simulink model "matrixconv1"  (Simulink 7.5)
settings: Solver=ode45  StartTime=0.0  StopTime=0.1  RelTol=1e-3
libraries: powerlib x46, powerlib_extras x4
settings Model: Creator=jeevitha  LastModifiedBy=Administrator
settings DebuggingCC: FcnCallInpInsideContextMsg=Enable All

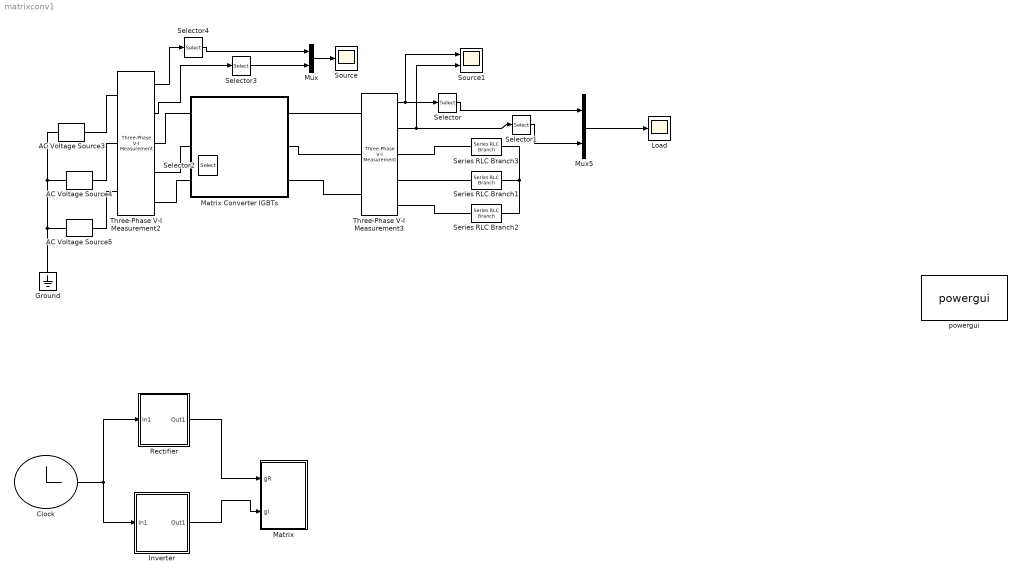
== system matrixconv1 ==
  AC Voltage Source3 : powerlib/Electrical Sources/AC Voltage Source  DialogController=POWERSYS.PowerSysDialog  SystemSampleTime=-1  Amplitude=230  Phase=0  Frequency=50  SampleTime=0  Measurements=None
  AC Voltage Source4 : powerlib/Electrical Sources/AC Voltage Source  DialogController=POWERSYS.PowerSysDialog  SystemSampleTime=-1  Amplitude=230  Phase=120  Frequency=50  SampleTime=0  Measurements=None
  AC Voltage Source5 : powerlib/Electrical Sources/AC Voltage Source  DialogController=POWERSYS.PowerSysDialog  SystemSampleTime=-1  Amplitude=230  Phase=-120  Frequency=50  SampleTime=0  Measurements=None
  Clock : Clock
  Ground : powerlib/Elements/Ground  DialogController=POWERSYS.PowerSysDialog  PhysicalDomain=powersysdomain  SubClassName=unknown  LeftPortType=p1  RightPortType=p1  LConnTagsString=a
  Inverter : Subsystem
  Load : Scope
      settings: TimeRange=0.012  YMin=-25  YMax=400  SaveName=vl
  Matrix : Subsystem
  Matrix Converter IGBTs : Subsystem
      mask Display:
      | plot([0 10],[0 0])
      | plot([0 10],[4 4])
      | plot([0 10],[8 8])
      | plot([10 11],[8 7],[11 12.5],[7 6.5],[12 13],[6 5])
      | plot([10 11]-4,[8 7],[11 12.5]-4,[7 6.5],[12 13]-4,[6 5])
      | plot([10 11]-8,[8 7],[11 12.5]-8,[7 6.5],[12 13]-8,[6 5])
      | plot([10 11],[8 7]-4,[11 12.5],[7 6.5]-4,[12 13],[6 5]-4)
      | plot([10 11]-4,[8 7]-4,[11 12.5]-4,[7 6.5]-4,[12 13]-4,[6 5]-4)
      | plot([10 11]-8,[8 7]-4,[11 12.5]-8,[7 6.5]-4,[12 13]-8,[6 5]-4)
      | plot([10 11],[8 7]-8,[11 12.5],[7 6.5]-8,[12 13],[6 5]-8)
      | plot([10 11]-4,[8 7]-8,[11 12.5]-4,[7 6.5]-8,[12 13]-4,[6 5]-8)
      | plot([10 11]-8,[8 7]-8,[11 12.5]-8,[7 6.5]-8,[12 13]-8,[6 5]-8)
      | plot([5 5],[-5 5])
      | plot([9 9],[-5 5])
      | plot([13 13],[-5 5])
      | plot(-2,-6,15,9)
      | plot([0 0],[-5 -2])
      | plot([0.5 0.5],[-5 -2])
      | plot([0.5 1.5],[-4 -5])
      | plot([0.5 1.5],[-3 -2])
      | plot([1.5 1.5],[-5 -6])
      | plot([1.5 1.5],[-2 -1])
      | plot([1 1.5],[-4.8 -5])
      | plot([1.3 1.5],[-4.4 -5])
      | plot([-0.5 0],[-5 -5])
  Mux : Mux  Inputs=2
  Mux5 : Mux  Inputs=2
  Rectifier : Subsystem
  Selector : Selector  InputPortWidth=3  IndexOptions=Index vector (dialog)  Indices=3  OutputSizes=1
  Selector1 : Selector  InputPortWidth=3  IndexOptions=Index vector (dialog)  Indices=3  OutputSizes=1
  Selector2 : Selector  InputPortWidth=3  IndexOptions=Index vector (dialog)  Indices=1  OutputSizes=1
  Selector3 : Selector  InputPortWidth=3  IndexOptions=Index vector (dialog)  Indices=1  OutputSizes=1
  Selector4 : Selector  InputPortWidth=3  IndexOptions=Index vector (dialog)  Indices=1  OutputSizes=1
  Series RLC Branch1 : powerlib/Elements/Series RLC Branch  DialogController=POWERSYS.PowerSysDialog  PhysicalDomain=powersysdomain  SubClassName=unknown  LeftPortType=p1  RightPortType=p1  LConnTagsString=__new0  RConnTagsString=__new0  BranchType=R  Resistance=2  Inductance=1e-3  SetiL0=off  InitialCurrent=0  Capacitance=[]  Setx0=off  InitialVoltage=0  Measurements=None
  Series RLC Branch2 : powerlib/Elements/Series RLC Branch  DialogController=POWERSYS.PowerSysDialog  PhysicalDomain=powersysdomain  SubClassName=unknown  LeftPortType=p1  RightPortType=p1  LConnTagsString=__new0  RConnTagsString=__new0  BranchType=R  Resistance=2  Inductance=1e-3  SetiL0=off  InitialCurrent=0  Capacitance=[]  Setx0=off  InitialVoltage=0  Measurements=None
  Series RLC Branch3 : powerlib/Elements/Series RLC Branch  DialogController=POWERSYS.PowerSysDialog  PhysicalDomain=powersysdomain  SubClassName=unknown  LeftPortType=p1  RightPortType=p1  LConnTagsString=__new0  RConnTagsString=__new0  BranchType=R  Resistance=2  Inductance=1e-3  SetiL0=off  InitialCurrent=0  Capacitance=[]  Setx0=off  InitialVoltage=0  Measurements=None
  Source : Scope
      settings: TimeRange=0.09  YMin=-100  YMax=100  SaveName=vl1
  Source1 : Scope  NumInputPorts=2
      settings: TimeRange=0.09  YMin=-100~-5  YMax=100~5  SaveName=vl2
  Three-Phase V-I Measurement2 : powerlib/Measurements/Three-Phase V-I Measurement  DialogController=POWERSYS.PowerSysDialog  SystemSampleTime=-1  VoltageMeasurement=phase-to-ground  SetLabelV=off  LabelV=Vabc  Vpu=off  VpuLL=off  CurrentMeasurement=yes  SetLabelI=off  LabelI=Iabc  Ipu=off  Pbase=100e6  Vbase=500e3  OutputType=Complex  PhasorSimulation=off  PSBequivalent=0
      link override Model/VI/Ia: GotoTag=LibraryTag_Ia
      link override Model/VI/Ib: GotoTag=LibraryTag_Ib
      link override Model/VI/Ic: GotoTag=LibraryTag_Ic
      link override Model/VI/Va: GotoTag=LibraryTag_Va
      link override Model/VI/Vb: GotoTag=LibraryTag_Vb
      link override Model/VI/Vc: GotoTag=LibraryTag_Vc
  Three-Phase V-I Measurement3 : powerlib/Measurements/Three-Phase V-I Measurement  DialogController=POWERSYS.PowerSysDialog  SystemSampleTime=-1  VoltageMeasurement=phase-to-phase  SetLabelV=off  LabelV=Vabc  Vpu=off  VpuLL=off  CurrentMeasurement=yes  SetLabelI=off  LabelI=Iabc  Ipu=off  Pbase=100e6  Vbase=500e3  OutputType=Complex  PhasorSimulation=off  PSBequivalent=0
      link override Model/VI/Ia: GotoTag=LibraryTag_Ia
      link override Model/VI/Ib: GotoTag=LibraryTag_Ib
      link override Model/VI/Ic: GotoTag=LibraryTag_Ic
      link override Model/VI/Va: GotoTag=LibraryTag_Va
      link override Model/VI/Vb: GotoTag=LibraryTag_Vb
      link override Model/VI/Vc: GotoTag=LibraryTag_Vc
  powergui : powerlib/powergui  Priority=1  SystemSampleTime=-1  SimulationMode=Discrete  SampleTime=((2e-4)/8)/100  frequency=60  SPID=off  DisableSnubberDevices=off  DisableRonSwitches=off  DisableVfSwitches=off  SwTol=0  Interpol=off  frequencyindice=0  echomessages=off  HookPort=off  DisplayEquations=off  FunctionMessages=off  EnableUseOfTLC=off  x0status=blocks  RestoreLinks=warning  ResistiveCurrentMeasurement=off  Frange=[0:2:500]  Ylog=off  Xlog=on  ShowGrid=off  save=off  variable=ZData  structure=ScopeData1  ZoomFFT=off  StartTime=0.02  cycles=1  DisplayStyle=3  fundamental=50  FreqAxis=off  MaxFrequency=1000  frequencyindicesteady=0  RmsSteady=2  display=off  Ts=0  methode=off
  wires:
  Clock/1 -> Rectifier/1(In1), Inverter/1(In1)
  Rectifier/1(Out1) -> Matrix/1(gR)
  Inverter/1(Out1) -> Matrix/2(gI)
  Three-Phase V-I Measurement3/1 -> Selector/1, Source1/1
  Three-Phase V-I Measurement3/2 -> Selector1/1, Source1/2
  Selector/1 -> Mux5/1
  Selector1/1 -> Mux5/2
  Mux5/1 -> Load/1
  Three-Phase V-I Measurement2/2 -> Selector3/1
  Three-Phase V-I Measurement2/1 -> Selector4/1
  Mux/1 -> Source/1
  Selector4/1 -> Mux/1
  Selector3/1 -> Mux/2
  connections:
  Series RLC Branch2/RConn1 -- Series RLC Branch3/RConn1 -- Series RLC Branch1/RConn1
  AC Voltage Source5/LConn1 -- Ground/LConn1 -- AC Voltage Source3/LConn1 -- AC Voltage Source4/LConn1
  Three-Phase V-I Measurement3/RConn1 -- Series RLC Branch3/LConn1
  Matrix Converter IGBTs/RConn1 -- Three-Phase V-I Measurement3/LConn1
  Matrix Converter IGBTs/RConn2 -- Three-Phase V-I Measurement3/LConn2
  Matrix Converter IGBTs/RConn3 -- Three-Phase V-I Measurement3/LConn3
  Three-Phase V-I Measurement3/RConn2 -- Series RLC Branch1/LConn1
  Three-Phase V-I Measurement3/RConn3 -- Series RLC Branch2/LConn1
  AC Voltage Source3/RConn1 -- Three-Phase V-I Measurement2/LConn1
  AC Voltage Source4/RConn1 -- Three-Phase V-I Measurement2/LConn2
  Three-Phase V-I Measurement2/LConn3 -- AC Voltage Source5/RConn1
  Three-Phase V-I Measurement2/RConn1 -- Matrix Converter IGBTs/LConn1
  Three-Phase V-I Measurement2/RConn2 -- Matrix Converter IGBTs/LConn2
  Three-Phase V-I Measurement2/RConn3 -- Matrix Converter IGBTs/LConn3

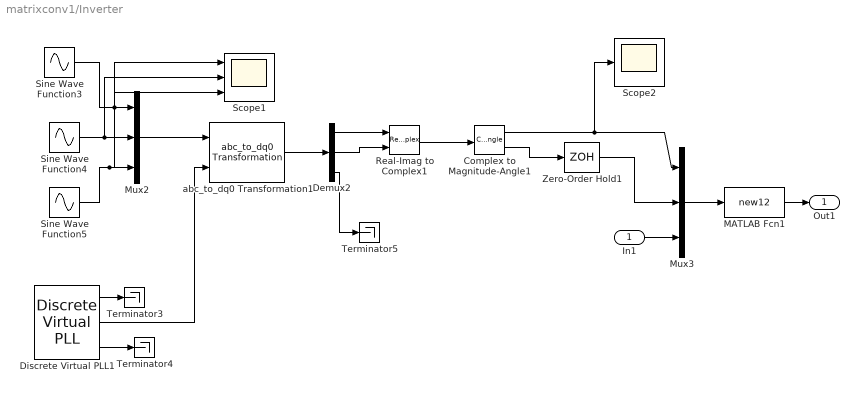
== system matrixconv1/Inverter ==
  In1 : Inport
  Complex to Magnitude-Angle1 : ComplexToMagnitudeAngle  SampleTime=((2e-4)/8)/100
  Demux2 : Demux  Outputs=3
  Discrete Virtual PLL1 : powerlib_extras/Discrete  Control Blocks/Discrete Virtual PLL  DialogController=POWERSYS.PowerSysDialog  SystemSampleTime=-1  Freq=25  Phase=0  Ts=((2e-4)/8)/100
  MATLAB Fcn1 : MATLABFcn  MATLABFcn=new12  OutputDimensions=6  SampleTime=((2e-4)/8)/100
  Mux2 : Mux  Inputs=3
  Mux3 : Mux  Inputs=3
  Real-Imag to Complex1 : RealImagToComplex  SampleTime=((2e-4)/8)/100
  Scope1 : Scope  NumInputPorts=3
      settings: YMin=0~175~-217  YMax=42.5~200~-199
  Scope2 : Scope
      settings: YMin=0  YMax=42.5  SaveName=ScopeData2
  Sine Wave Function3 : Sin  Amplitude=230  Bias=0  Frequency=2*pi*25  Phase=-(pi/6)  Samples=10  Offset=0
  Sine Wave Function4 : Sin  Amplitude=230  Bias=0  Frequency=2*pi*25  Phase=(2*pi/3)-(pi/6)  Samples=10  Offset=0
  Sine Wave Function5 : Sin  Amplitude=230  Bias=0  Frequency=2*pi*25  Phase=(4*pi/3)-(pi/6)  Samples=10  Offset=0
  Terminator3 : Terminator
  Terminator4 : Terminator
  Terminator5 : Terminator
  Zero-Order Hold1 : ZeroOrderHold  SampleTime=.0001005
  abc_to_dq0 Transformation1 : powerlib_extras/Measurements/abc_to_dq0 Transformation  DialogController=POWERSYS.PowerSysDialog  SystemSampleTime=-1
  Out1 : Outport
  wires:
  Discrete Virtual PLL1/1 -> Terminator3/1
  Discrete Virtual PLL1/3 -> Terminator4/1
  Sine Wave Function3/1 -> Mux2/1, Scope1/1
  Sine Wave Function4/1 -> Mux2/2, Scope1/2
  Sine Wave Function5/1 -> Mux2/3, Scope1/3
  Mux2/1 -> abc_to_dq0 Transformation1/1
  Discrete Virtual PLL1/2 -> abc_to_dq0 Transformation1/2
  abc_to_dq0 Transformation1/1 -> Demux2/1
  Demux2/3 -> Terminator5/1
  Demux2/1 -> Real-Imag to Complex1/1
  Demux2/2 -> Real-Imag to Complex1/2
  Real-Imag to Complex1/1 -> Complex to Magnitude-Angle1/1
  Complex to Magnitude-Angle1/2 -> Zero-Order Hold1/1
  Complex to Magnitude-Angle1/1 -> Mux3/1, Scope2/1
  Zero-Order Hold1/1 -> Mux3/2
  Mux3/1 -> MATLAB Fcn1/1
  In1/1 -> Mux3/3
  MATLAB Fcn1/1 -> Out1/1

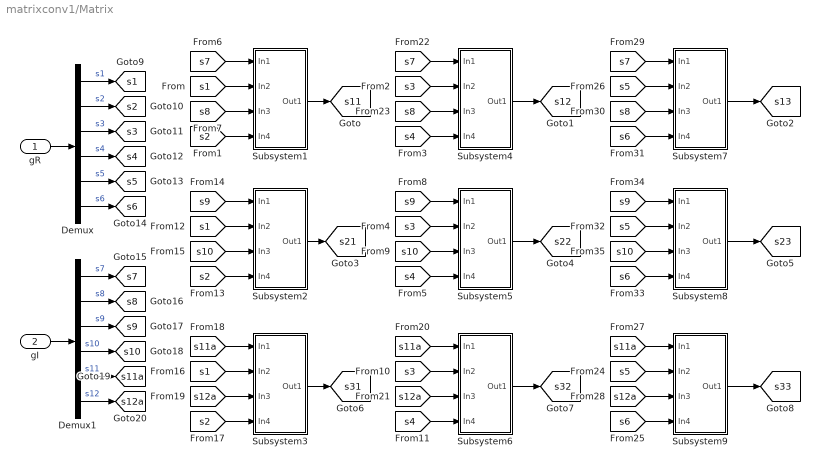
== system matrixconv1/Matrix ==
  gR : Inport
  gI : Inport  Port=2
  Demux : Demux  Outputs=6
  Demux1 : Demux  Outputs=6
  Subsystem1 : Subsystem
  Subsystem2 : Subsystem
  Subsystem3 : Subsystem
  Subsystem4 : Subsystem
  Subsystem5 : Subsystem
  Subsystem6 : Subsystem
  Subsystem7 : Subsystem
  Subsystem8 : Subsystem
  Subsystem9 : Subsystem
  tag scope: s10=global, s11=global, s11a=global, s12=global, s12a=global, s13=global, s1=global, s21=global, s22=global, s23=global, s2=global, s31=global, s32=global, s33=global, s3=global, s4=global, s5=global, s6=global, s7=global, s8=global, s9=global
  wires:
  Demux/4 -> [s4]  "s4"
  gR/1 -> Demux/1
  gI/1 -> Demux1/1
  Demux/1 -> [s1]  "s1"
  Demux1/1 -> [s7]  "s7"
  Demux/2 -> [s2]  "s2"
  Demux/3 -> [s3]  "s3"
  Demux/5 -> [s5]  "s5"
  Demux/6 -> [s6]  "s6"
  [s7] -> Subsystem1/1(In1)
  [s1] -> Subsystem1/2(In2)
  [s8] -> Subsystem1/3(In3)
  [s2] -> Subsystem1/4(In4)
  [s9] -> Subsystem2/1(In1)
  [s1] -> Subsystem2/2(In2)
  [s10] -> Subsystem2/3(In3)
  [s2] -> Subsystem2/4(In4)
  [s11a] -> Subsystem3/1(In1)
  [s1] -> Subsystem3/2(In2)
  [s12a] -> Subsystem3/3(In3)
  [s2] -> Subsystem3/4(In4)
  [s7] -> Subsystem4/1(In1)
  [s3] -> Subsystem4/2(In2)
  [s8] -> Subsystem4/3(In3)
  [s4] -> Subsystem4/4(In4)
  [s9] -> Subsystem5/1(In1)
  [s3] -> Subsystem5/2(In2)
  [s10] -> Subsystem5/3(In3)
  [s4] -> Subsystem5/4(In4)
  [s11a] -> Subsystem6/1(In1)
  [s3] -> Subsystem6/2(In2)
  [s12a] -> Subsystem6/3(In3)
  [s4] -> Subsystem6/4(In4)
  [s7] -> Subsystem7/1(In1)
  [s5] -> Subsystem7/2(In2)
  [s8] -> Subsystem7/3(In3)
  [s6] -> Subsystem7/4(In4)
  [s9] -> Subsystem8/1(In1)
  [s5] -> Subsystem8/2(In2)
  [s10] -> Subsystem8/3(In3)
  [s6] -> Subsystem8/4(In4)
  [s11a] -> Subsystem9/1(In1)
  [s5] -> Subsystem9/2(In2)
  [s12a] -> Subsystem9/3(In3)
  [s6] -> Subsystem9/4(In4)
  Subsystem1/1(Out1) -> [s11]
  Subsystem4/1(Out1) -> [s12]
  Subsystem7/1(Out1) -> [s13]
  Subsystem2/1(Out1) -> [s21]
  Subsystem5/1(Out1) -> [s22]
  Subsystem8/1(Out1) -> [s23]
  Subsystem3/1(Out1) -> [s31]
  Subsystem6/1(Out1) -> [s32]
  Subsystem9/1(Out1) -> [s33]
  Demux1/2 -> [s8]  "s8"
  Demux1/3 -> [s9]  "s9"
  Demux1/4 -> [s10]  "s10"
  Demux1/5 -> [s11a]  "s11"
  Demux1/6 -> [s12a]  "s12"

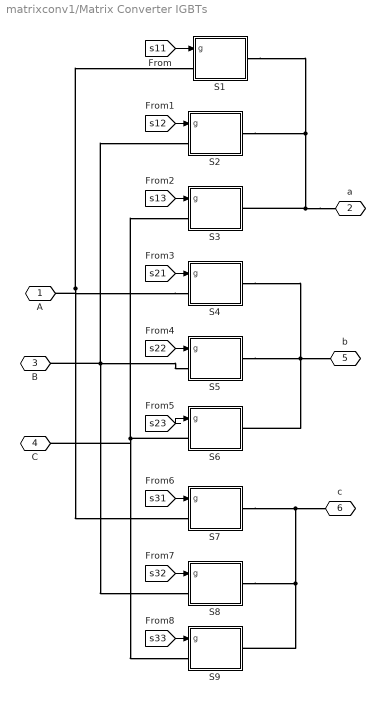
== system matrixconv1/Matrix Converter IGBTs ==
  S1 : Subsystem
  S2 : Subsystem
  S3 : Subsystem
  S4 : Subsystem
  S5 : Subsystem
  S6 : Subsystem
  S7 : Subsystem
  S8 : Subsystem
  S9 : Subsystem
  A : PMIOPort  Port=1  Side=Left
  a : PMIOPort  Port=2  Side=Right
  B : PMIOPort  Port=3  Side=Left
  C : PMIOPort  Port=4  Side=Left
  b : PMIOPort  Port=5  Side=Right
  c : PMIOPort  Port=6  Side=Right
  wires:
  [s11] -> S1/1(g)
  [s12] -> S2/1(g)
  [s13] -> S3/1(g)
  [s21] -> S4/1(g)
  [s22] -> S5/1(g)
  [s23] -> S6/1(g)
  [s31] -> S7/1(g)
  [s32] -> S8/1(g)
  [s33] -> S9/1(g)
  connections:
  S4/LConn1 -- A/RConn1 -- S1/LConn1 -- S7/LConn1
  a/RConn1 -- S2/RConn1 -- S1/RConn1 -- S3/RConn1
  S5/LConn1 -- S2/LConn1 -- B/RConn1 -- S8/LConn1
  S6/LConn1 -- S3/LConn1 -- C/RConn1 -- S9/LConn1
  S5/RConn1 -- S4/RConn1 -- b/RConn1 -- S6/RConn1
  S8/RConn1 -- S7/RConn1 -- c/RConn1 -- S9/RConn1

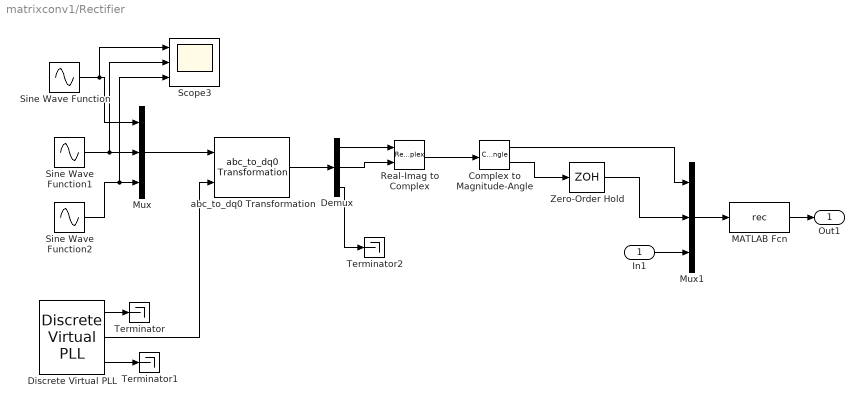
== system matrixconv1/Rectifier ==
  In1 : Inport
  Complex to Magnitude-Angle : ComplexToMagnitudeAngle  SampleTime=((2e-4)/8)/100
  Demux : Demux  Outputs=3
  Discrete Virtual PLL : powerlib_extras/Discrete  Control Blocks/Discrete Virtual PLL  DialogController=POWERSYS.PowerSysDialog  SystemSampleTime=-1  Freq=25  Phase=0  Ts=((2e-4)/8)/100
  MATLAB Fcn : MATLABFcn  MATLABFcn=rec  OutputDimensions=6  SampleTime=((2e-4)/8)/100
  Mux : Mux  Inputs=3
  Mux1 : Mux  Inputs=3
  Real-Imag to Complex : RealImagToComplex  SampleTime=((2e-4)/8)/100
  Scope3 : Scope  NumInputPorts=3
      settings: YMin=-182.5~213~-82.5  YMax=-145~227~-32.5
  Sine Wave Function : Sin  Amplitude=230  Bias=0  Frequency=2*pi*25  Phase=+(pi/6)  Samples=10  Offset=0
  Sine Wave Function1 : Sin  Amplitude=230  Bias=0  Frequency=2*pi*25  Phase=(2*pi/3)+(pi/6)  Samples=10  Offset=0
  Sine Wave Function2 : Sin  Amplitude=230  Bias=0  Frequency=2*pi*25  Phase=(4*pi/3)+(pi/6)  Samples=10  Offset=0
  Terminator : Terminator
  Terminator1 : Terminator
  Terminator2 : Terminator
  Zero-Order Hold : ZeroOrderHold  SampleTime=.0001005
  abc_to_dq0 Transformation : powerlib_extras/Measurements/abc_to_dq0 Transformation  DialogController=POWERSYS.PowerSysDialog  SystemSampleTime=-1
  Out1 : Outport
  wires:
  Discrete Virtual PLL/1 -> Terminator/1
  Discrete Virtual PLL/3 -> Terminator1/1
  Sine Wave Function/1 -> Mux/1, Scope3/1
  Sine Wave Function1/1 -> Mux/2, Scope3/2
  Sine Wave Function2/1 -> Mux/3, Scope3/3
  Mux/1 -> abc_to_dq0 Transformation/1
  Discrete Virtual PLL/2 -> abc_to_dq0 Transformation/2
  abc_to_dq0 Transformation/1 -> Demux/1
  Demux/3 -> Terminator2/1
  Demux/1 -> Real-Imag to Complex/1
  Demux/2 -> Real-Imag to Complex/2
  Real-Imag to Complex/1 -> Complex to Magnitude-Angle/1
  Complex to Magnitude-Angle/2 -> Zero-Order Hold/1
  Complex to Magnitude-Angle/1 -> Mux1/1
  Zero-Order Hold/1 -> Mux1/2
  Mux1/1 -> MATLAB Fcn/1
  In1/1 -> Mux1/3
  MATLAB Fcn/1 -> Out1/1

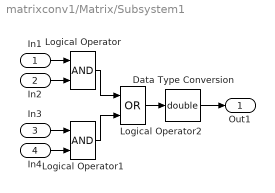
== system matrixconv1/Matrix/Subsystem1 ==
  In1 : Inport
  In2 : Inport  Port=2
  In3 : Inport  Port=3
  In4 : Inport  Port=4
  Data Type Conversion : DataTypeConversion  OutDataTypeMode=double  OutDataTypeStr=double
  Logical Operator : Logic  AllPortsSameDT=off  OutDataTypeMode=boolean  OutDataTypeStr=boolean
  Logical Operator1 : Logic  AllPortsSameDT=off  OutDataTypeMode=boolean  OutDataTypeStr=boolean
  Logical Operator2 : Logic  Operator=OR  AllPortsSameDT=off  OutDataTypeMode=boolean  OutDataTypeStr=boolean
  Out1 : Outport
  wires:
  In4/1 -> Logical Operator1/2
  In3/1 -> Logical Operator1/1
  Logical Operator2/1 -> Data Type Conversion/1
  In2/1 -> Logical Operator/2
  In1/1 -> Logical Operator/1
  Logical Operator1/1 -> Logical Operator2/2
  Logical Operator/1 -> Logical Operator2/1
  Data Type Conversion/1 -> Out1/1

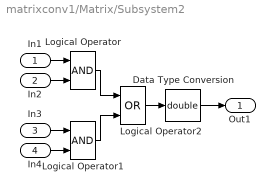
== system matrixconv1/Matrix/Subsystem2 ==
  In1 : Inport
  In2 : Inport  Port=2
  In3 : Inport  Port=3
  In4 : Inport  Port=4
  Data Type Conversion : DataTypeConversion  OutDataTypeMode=double  OutDataTypeStr=double
  Logical Operator : Logic  AllPortsSameDT=off  OutDataTypeMode=boolean  OutDataTypeStr=boolean
  Logical Operator1 : Logic  AllPortsSameDT=off  OutDataTypeMode=boolean  OutDataTypeStr=boolean
  Logical Operator2 : Logic  Operator=OR  AllPortsSameDT=off  OutDataTypeMode=boolean  OutDataTypeStr=boolean
  Out1 : Outport
  wires:
  In4/1 -> Logical Operator1/2
  In3/1 -> Logical Operator1/1
  Logical Operator2/1 -> Data Type Conversion/1
  In2/1 -> Logical Operator/2
  In1/1 -> Logical Operator/1
  Logical Operator1/1 -> Logical Operator2/2
  Logical Operator/1 -> Logical Operator2/1
  Data Type Conversion/1 -> Out1/1

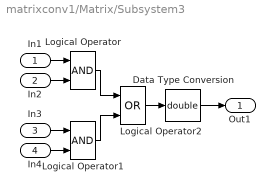
== system matrixconv1/Matrix/Subsystem3 ==
  In1 : Inport
  In2 : Inport  Port=2
  In3 : Inport  Port=3
  In4 : Inport  Port=4
  Data Type Conversion : DataTypeConversion  OutDataTypeMode=double  OutDataTypeStr=double
  Logical Operator : Logic  AllPortsSameDT=off  OutDataTypeMode=boolean  OutDataTypeStr=boolean
  Logical Operator1 : Logic  AllPortsSameDT=off  OutDataTypeMode=boolean  OutDataTypeStr=boolean
  Logical Operator2 : Logic  Operator=OR  AllPortsSameDT=off  OutDataTypeMode=boolean  OutDataTypeStr=boolean
  Out1 : Outport
  wires:
  In4/1 -> Logical Operator1/2
  In3/1 -> Logical Operator1/1
  Logical Operator2/1 -> Data Type Conversion/1
  In2/1 -> Logical Operator/2
  In1/1 -> Logical Operator/1
  Logical Operator1/1 -> Logical Operator2/2
  Logical Operator/1 -> Logical Operator2/1
  Data Type Conversion/1 -> Out1/1

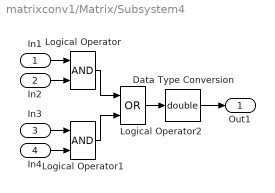
== system matrixconv1/Matrix/Subsystem4 ==
  In1 : Inport
  In2 : Inport  Port=2
  In3 : Inport  Port=3
  In4 : Inport  Port=4
  Data Type Conversion : DataTypeConversion  OutDataTypeMode=double  OutDataTypeStr=double
  Logical Operator : Logic  AllPortsSameDT=off  OutDataTypeMode=boolean  OutDataTypeStr=boolean
  Logical Operator1 : Logic  AllPortsSameDT=off  OutDataTypeMode=boolean  OutDataTypeStr=boolean
  Logical Operator2 : Logic  Operator=OR  AllPortsSameDT=off  OutDataTypeMode=boolean  OutDataTypeStr=boolean
  Out1 : Outport
  wires:
  In4/1 -> Logical Operator1/2
  In3/1 -> Logical Operator1/1
  Logical Operator2/1 -> Data Type Conversion/1
  In2/1 -> Logical Operator/2
  In1/1 -> Logical Operator/1
  Logical Operator1/1 -> Logical Operator2/2
  Logical Operator/1 -> Logical Operator2/1
  Data Type Conversion/1 -> Out1/1

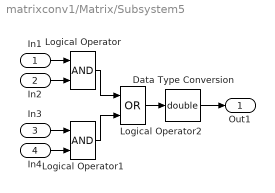
== system matrixconv1/Matrix/Subsystem5 ==
  In1 : Inport
  In2 : Inport  Port=2
  In3 : Inport  Port=3
  In4 : Inport  Port=4
  Data Type Conversion : DataTypeConversion  OutDataTypeMode=double  OutDataTypeStr=double
  Logical Operator : Logic  AllPortsSameDT=off  OutDataTypeMode=boolean  OutDataTypeStr=boolean
  Logical Operator1 : Logic  AllPortsSameDT=off  OutDataTypeMode=boolean  OutDataTypeStr=boolean
  Logical Operator2 : Logic  Operator=OR  AllPortsSameDT=off  OutDataTypeMode=boolean  OutDataTypeStr=boolean
  Out1 : Outport
  wires:
  In4/1 -> Logical Operator1/2
  In3/1 -> Logical Operator1/1
  Logical Operator2/1 -> Data Type Conversion/1
  In2/1 -> Logical Operator/2
  In1/1 -> Logical Operator/1
  Logical Operator1/1 -> Logical Operator2/2
  Logical Operator/1 -> Logical Operator2/1
  Data Type Conversion/1 -> Out1/1

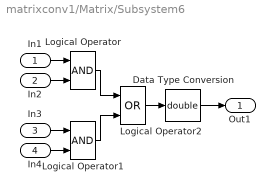
== system matrixconv1/Matrix/Subsystem6 ==
  In1 : Inport
  In2 : Inport  Port=2
  In3 : Inport  Port=3
  In4 : Inport  Port=4
  Data Type Conversion : DataTypeConversion  OutDataTypeMode=double  OutDataTypeStr=double
  Logical Operator : Logic  AllPortsSameDT=off  OutDataTypeMode=boolean  OutDataTypeStr=boolean
  Logical Operator1 : Logic  AllPortsSameDT=off  OutDataTypeMode=boolean  OutDataTypeStr=boolean
  Logical Operator2 : Logic  Operator=OR  AllPortsSameDT=off  OutDataTypeMode=boolean  OutDataTypeStr=boolean
  Out1 : Outport
  wires:
  In4/1 -> Logical Operator1/2
  In3/1 -> Logical Operator1/1
  Logical Operator2/1 -> Data Type Conversion/1
  In2/1 -> Logical Operator/2
  In1/1 -> Logical Operator/1
  Logical Operator1/1 -> Logical Operator2/2
  Logical Operator/1 -> Logical Operator2/1
  Data Type Conversion/1 -> Out1/1

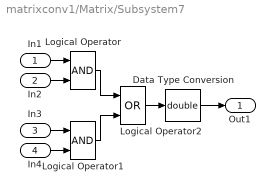
== system matrixconv1/Matrix/Subsystem7 ==
  In1 : Inport
  In2 : Inport  Port=2
  In3 : Inport  Port=3
  In4 : Inport  Port=4
  Data Type Conversion : DataTypeConversion  OutDataTypeMode=double  OutDataTypeStr=double
  Logical Operator : Logic  AllPortsSameDT=off  OutDataTypeMode=boolean  OutDataTypeStr=boolean
  Logical Operator1 : Logic  AllPortsSameDT=off  OutDataTypeMode=boolean  OutDataTypeStr=boolean
  Logical Operator2 : Logic  Operator=OR  AllPortsSameDT=off  OutDataTypeMode=boolean  OutDataTypeStr=boolean
  Out1 : Outport
  wires:
  In4/1 -> Logical Operator1/2
  In3/1 -> Logical Operator1/1
  Logical Operator2/1 -> Data Type Conversion/1
  In2/1 -> Logical Operator/2
  In1/1 -> Logical Operator/1
  Logical Operator1/1 -> Logical Operator2/2
  Logical Operator/1 -> Logical Operator2/1
  Data Type Conversion/1 -> Out1/1

== system matrixconv1/Matrix/Subsystem8 ==
  In1 : Inport
  In2 : Inport  Port=2
  In3 : Inport  Port=3
  In4 : Inport  Port=4
  Data Type Conversion : DataTypeConversion  OutDataTypeMode=double  OutDataTypeStr=double
  Logical Operator : Logic  AllPortsSameDT=off  OutDataTypeMode=boolean  OutDataTypeStr=boolean
  Logical Operator1 : Logic  AllPortsSameDT=off  OutDataTypeMode=boolean  OutDataTypeStr=boolean
  Logical Operator2 : Logic  Operator=OR  AllPortsSameDT=off  OutDataTypeMode=boolean  OutDataTypeStr=boolean
  Out1 : Outport
  wires:
  In4/1 -> Logical Operator1/2
  In3/1 -> Logical Operator1/1
  Logical Operator2/1 -> Data Type Conversion/1
  In2/1 -> Logical Operator/2
  In1/1 -> Logical Operator/1
  Logical Operator1/1 -> Logical Operator2/2
  Logical Operator/1 -> Logical Operator2/1
  Data Type Conversion/1 -> Out1/1

== system matrixconv1/Matrix/Subsystem9 ==
  In1 : Inport
  In2 : Inport  Port=2
  In3 : Inport  Port=3
  In4 : Inport  Port=4
  Data Type Conversion : DataTypeConversion  OutDataTypeMode=double  OutDataTypeStr=double
  Logical Operator : Logic  AllPortsSameDT=off  OutDataTypeMode=boolean  OutDataTypeStr=boolean
  Logical Operator1 : Logic  AllPortsSameDT=off  OutDataTypeMode=boolean  OutDataTypeStr=boolean
  Logical Operator2 : Logic  Operator=OR  AllPortsSameDT=off  OutDataTypeMode=boolean  OutDataTypeStr=boolean
  Out1 : Outport
  wires:
  In4/1 -> Logical Operator1/2
  In3/1 -> Logical Operator1/1
  Logical Operator2/1 -> Data Type Conversion/1
  In2/1 -> Logical Operator/2
  In1/1 -> Logical Operator/1
  Logical Operator1/1 -> Logical Operator2/2
  Logical Operator/1 -> Logical Operator2/1
  Data Type Conversion/1 -> Out1/1

== system matrixconv1/Matrix Converter IGBTs/S1 ==
  g : Inport
  Diode : powerlib/Power Electronics/Diode  DialogController=POWERSYS.PowerSysDialog  SystemSampleTime=-1  Ron=0.001  Lon=0  Vf=0  IC=0  UseSnubber=off  Rs=1e4  Cs=250e-9  Measurements=off
  Diode1 : powerlib/Power Electronics/Diode  DialogController=POWERSYS.PowerSysDialog  SystemSampleTime=-1  Ron=0.001  Lon=0  Vf=0  IC=0  UseSnubber=off  Rs=1e4  Cs=250e-9  Measurements=off
  IGBT1 : powerlib/Power Electronics/IGBT  DialogController=POWERSYS.PowerSysDialog  SystemSampleTime=-1  Ron=0.001  Lon=0  Vf=1  Tf=1e-6  Tt=2e-6  IC=0  Rs=1e5  Cs=inf  Measurements=off
  IGBT2 : powerlib/Power Electronics/IGBT  DialogController=POWERSYS.PowerSysDialog  SystemSampleTime=-1  Ron=0.001  Lon=0  Vf=1  Tf=1e-6  Tt=2e-6  IC=0  Rs=1e5  Cs=inf  Measurements=off
  + : PMIOPort  Port=1  Side=Left
  - : PMIOPort  Port=2  Side=Right
  wires:
  g/1 -> IGBT1/1, IGBT2/1
  connections:
  Diode1/LConn1 -- Diode/LConn1 -- IGBT1/RConn1 -- IGBT2/RConn1
  -/RConn1 -- Diode1/RConn1 -- IGBT1/LConn1
  +/RConn1 -- Diode/RConn1 -- IGBT2/LConn1

== system matrixconv1/Matrix Converter IGBTs/S2 ==
  g : Inport
  Diode : powerlib/Power Electronics/Diode  DialogController=POWERSYS.PowerSysDialog  SystemSampleTime=-1  Ron=0.001  Lon=0  Vf=0  IC=0  UseSnubber=off  Rs=1e4  Cs=250e-9  Measurements=off
  Diode1 : powerlib/Power Electronics/Diode  DialogController=POWERSYS.PowerSysDialog  SystemSampleTime=-1  Ron=0.001  Lon=0  Vf=0  IC=0  UseSnubber=off  Rs=1e4  Cs=250e-9  Measurements=off
  IGBT1 : powerlib/Power Electronics/IGBT  DialogController=POWERSYS.PowerSysDialog  SystemSampleTime=-1  Ron=0.001  Lon=0  Vf=1  Tf=1e-6  Tt=2e-6  IC=0  Rs=1e5  Cs=inf  Measurements=off
  IGBT2 : powerlib/Power Electronics/IGBT  DialogController=POWERSYS.PowerSysDialog  SystemSampleTime=-1  Ron=0.001  Lon=0  Vf=1  Tf=1e-6  Tt=2e-6  IC=0  Rs=1e5  Cs=inf  Measurements=off
  + : PMIOPort  Port=1  Side=Left
  - : PMIOPort  Port=2  Side=Right
  wires:
  g/1 -> IGBT2/1, IGBT1/1
  connections:
  +/RConn1 -- IGBT2/LConn1 -- Diode/RConn1
  -/RConn1 -- IGBT1/LConn1 -- Diode1/RConn1
  Diode/LConn1 -- IGBT2/RConn1 -- IGBT1/RConn1 -- Diode1/LConn1

== system matrixconv1/Matrix Converter IGBTs/S3 ==
  g : Inport
  Diode : powerlib/Power Electronics/Diode  DialogController=POWERSYS.PowerSysDialog  SystemSampleTime=-1  Ron=0.001  Lon=0  Vf=0  IC=0  UseSnubber=off  Rs=1e4  Cs=250e-9  Measurements=off
  Diode1 : powerlib/Power Electronics/Diode  DialogController=POWERSYS.PowerSysDialog  SystemSampleTime=-1  Ron=0.001  Lon=0  Vf=0  IC=0  UseSnubber=off  Rs=1e4  Cs=250e-9  Measurements=off
  IGBT1 : powerlib/Power Electronics/IGBT  DialogController=POWERSYS.PowerSysDialog  SystemSampleTime=-1  Ron=0.001  Lon=0  Vf=1  Tf=1e-6  Tt=2e-6  IC=0  Rs=1e5  Cs=inf  Measurements=off
  IGBT2 : powerlib/Power Electronics/IGBT  DialogController=POWERSYS.PowerSysDialog  SystemSampleTime=-1  Ron=0.001  Lon=0  Vf=1  Tf=1e-6  Tt=2e-6  IC=0  Rs=1e5  Cs=inf  Measurements=off
  + : PMIOPort  Port=1  Side=Left
  - : PMIOPort  Port=2  Side=Right
  wires:
  g/1 -> IGBT1/1, IGBT2/1
  connections:
  Diode1/LConn1 -- IGBT1/RConn1 -- IGBT2/RConn1 -- Diode/LConn1
  Diode1/RConn1 -- IGBT1/LConn1 -- -/RConn1
  Diode/RConn1 -- IGBT2/LConn1 -- +/RConn1

== system matrixconv1/Matrix Converter IGBTs/S4 ==
  g : Inport
  Diode : powerlib/Power Electronics/Diode  DialogController=POWERSYS.PowerSysDialog  SystemSampleTime=-1  Ron=0.001  Lon=0  Vf=0  IC=0  UseSnubber=off  Rs=1e4  Cs=250e-9  Measurements=off
  Diode1 : powerlib/Power Electronics/Diode  DialogController=POWERSYS.PowerSysDialog  SystemSampleTime=-1  Ron=0.001  Lon=0  Vf=0  IC=0  UseSnubber=off  Rs=1e4  Cs=250e-9  Measurements=off
  IGBT1 : powerlib/Power Electronics/IGBT  DialogController=POWERSYS.PowerSysDialog  SystemSampleTime=-1  Ron=0.001  Lon=0  Vf=1  Tf=1e-6  Tt=2e-6  IC=0  Rs=1e5  Cs=inf  Measurements=off
  IGBT2 : powerlib/Power Electronics/IGBT  DialogController=POWERSYS.PowerSysDialog  SystemSampleTime=-1  Ron=0.001  Lon=0  Vf=1  Tf=1e-6  Tt=2e-6  IC=0  Rs=1e5  Cs=inf  Measurements=off
  + : PMIOPort  Port=1  Side=Left
  - : PMIOPort  Port=2  Side=Right
  wires:
  g/1 -> IGBT2/1, IGBT1/1
  connections:
  +/RConn1 -- IGBT2/LConn1 -- Diode/RConn1
  -/RConn1 -- IGBT1/LConn1 -- Diode1/RConn1
  Diode/LConn1 -- IGBT2/RConn1 -- IGBT1/RConn1 -- Diode1/LConn1

== system matrixconv1/Matrix Converter IGBTs/S5 ==
  g : Inport
  Diode : powerlib/Power Electronics/Diode  DialogController=POWERSYS.PowerSysDialog  SystemSampleTime=-1  Ron=0.001  Lon=0  Vf=0  IC=0  UseSnubber=off  Rs=1e4  Cs=250e-9  Measurements=off
  Diode1 : powerlib/Power Electronics/Diode  DialogController=POWERSYS.PowerSysDialog  SystemSampleTime=-1  Ron=0.001  Lon=0  Vf=0  IC=0  UseSnubber=off  Rs=1e4  Cs=250e-9  Measurements=off
  IGBT1 : powerlib/Power Electronics/IGBT  DialogController=POWERSYS.PowerSysDialog  SystemSampleTime=-1  Ron=0.001  Lon=0  Vf=1  Tf=1e-6  Tt=2e-6  IC=0  Rs=1e5  Cs=inf  Measurements=off
  IGBT2 : powerlib/Power Electronics/IGBT  DialogController=POWERSYS.PowerSysDialog  SystemSampleTime=-1  Ron=0.001  Lon=0  Vf=1  Tf=1e-6  Tt=2e-6  IC=0  Rs=1e5  Cs=inf  Measurements=off
  + : PMIOPort  Port=1  Side=Left
  - : PMIOPort  Port=2  Side=Right
  wires:
  g/1 -> IGBT1/1, IGBT2/1
  connections:
  Diode1/LConn1 -- IGBT1/RConn1 -- IGBT2/RConn1 -- Diode/LConn1
  Diode1/RConn1 -- IGBT1/LConn1 -- -/RConn1
  Diode/RConn1 -- IGBT2/LConn1 -- +/RConn1

== system matrixconv1/Matrix Converter IGBTs/S6 ==
  g : Inport
  Diode : powerlib/Power Electronics/Diode  DialogController=POWERSYS.PowerSysDialog  SystemSampleTime=-1  Ron=0.001  Lon=0  Vf=0  IC=0  UseSnubber=off  Rs=1e4  Cs=250e-9  Measurements=off
  Diode1 : powerlib/Power Electronics/Diode  DialogController=POWERSYS.PowerSysDialog  SystemSampleTime=-1  Ron=0.001  Lon=0  Vf=0  IC=0  UseSnubber=off  Rs=1e4  Cs=250e-9  Measurements=off
  IGBT1 : powerlib/Power Electronics/IGBT  DialogController=POWERSYS.PowerSysDialog  SystemSampleTime=-1  Ron=0.001  Lon=0  Vf=1  Tf=1e-6  Tt=2e-6  IC=0  Rs=1e5  Cs=inf  Measurements=off
  IGBT2 : powerlib/Power Electronics/IGBT  DialogController=POWERSYS.PowerSysDialog  SystemSampleTime=-1  Ron=0.001  Lon=0  Vf=1  Tf=1e-6  Tt=2e-6  IC=0  Rs=1e5  Cs=inf  Measurements=off
  + : PMIOPort  Port=1  Side=Left
  - : PMIOPort  Port=2  Side=Right
  wires:
  g/1 -> IGBT2/1, IGBT1/1
  connections:
  +/RConn1 -- IGBT2/LConn1 -- Diode/RConn1
  -/RConn1 -- IGBT1/LConn1 -- Diode1/RConn1
  Diode/LConn1 -- IGBT2/RConn1 -- IGBT1/RConn1 -- Diode1/LConn1

== system matrixconv1/Matrix Converter IGBTs/S7 ==
  g : Inport
  Diode : powerlib/Power Electronics/Diode  DialogController=POWERSYS.PowerSysDialog  SystemSampleTime=-1  Ron=0.001  Lon=0  Vf=0  IC=0  UseSnubber=off  Rs=1e4  Cs=250e-9  Measurements=off
  Diode1 : powerlib/Power Electronics/Diode  DialogController=POWERSYS.PowerSysDialog  SystemSampleTime=-1  Ron=0.001  Lon=0  Vf=0  IC=0  UseSnubber=off  Rs=1e4  Cs=250e-9  Measurements=off
  IGBT1 : powerlib/Power Electronics/IGBT  DialogController=POWERSYS.PowerSysDialog  SystemSampleTime=-1  Ron=0.001  Lon=0  Vf=1  Tf=1e-6  Tt=2e-6  IC=0  Rs=1e5  Cs=inf  Measurements=off
  IGBT2 : powerlib/Power Electronics/IGBT  DialogController=POWERSYS.PowerSysDialog  SystemSampleTime=-1  Ron=0.001  Lon=0  Vf=1  Tf=1e-6  Tt=2e-6  IC=0  Rs=1e5  Cs=inf  Measurements=off
  + : PMIOPort  Port=1  Side=Left
  - : PMIOPort  Port=2  Side=Right
  wires:
  g/1 -> IGBT1/1, IGBT2/1
  connections:
  Diode1/LConn1 -- IGBT1/RConn1 -- IGBT2/RConn1 -- Diode/LConn1
  Diode1/RConn1 -- IGBT1/LConn1 -- -/RConn1
  Diode/RConn1 -- IGBT2/LConn1 -- +/RConn1

== system matrixconv1/Matrix Converter IGBTs/S8 ==
  g : Inport
  Diode : powerlib/Power Electronics/Diode  DialogController=POWERSYS.PowerSysDialog  SystemSampleTime=-1  Ron=0.001  Lon=0  Vf=0  IC=0  UseSnubber=off  Rs=1e4  Cs=250e-9  Measurements=off
  Diode1 : powerlib/Power Electronics/Diode  DialogController=POWERSYS.PowerSysDialog  SystemSampleTime=-1  Ron=0.001  Lon=0  Vf=0  IC=0  UseSnubber=off  Rs=1e4  Cs=250e-9  Measurements=off
  IGBT1 : powerlib/Power Electronics/IGBT  DialogController=POWERSYS.PowerSysDialog  SystemSampleTime=-1  Ron=0.001  Lon=0  Vf=1  Tf=1e-6  Tt=2e-6  IC=0  Rs=1e5  Cs=inf  Measurements=off
  IGBT2 : powerlib/Power Electronics/IGBT  DialogController=POWERSYS.PowerSysDialog  SystemSampleTime=-1  Ron=0.001  Lon=0  Vf=1  Tf=1e-6  Tt=2e-6  IC=0  Rs=1e5  Cs=inf  Measurements=off
  + : PMIOPort  Port=1  Side=Left
  - : PMIOPort  Port=2  Side=Right
  wires:
  g/1 -> IGBT2/1, IGBT1/1
  connections:
  +/RConn1 -- IGBT2/LConn1 -- Diode/RConn1
  -/RConn1 -- IGBT1/LConn1 -- Diode1/RConn1
  Diode/LConn1 -- IGBT2/RConn1 -- IGBT1/RConn1 -- Diode1/LConn1

== system matrixconv1/Matrix Converter IGBTs/S9 ==
  g : Inport
  Diode : powerlib/Power Electronics/Diode  DialogController=POWERSYS.PowerSysDialog  SystemSampleTime=-1  Ron=0.001  Lon=0  Vf=0  IC=0  UseSnubber=off  Rs=1e4  Cs=250e-9  Measurements=off
  Diode1 : powerlib/Power Electronics/Diode  DialogController=POWERSYS.PowerSysDialog  SystemSampleTime=-1  Ron=0.001  Lon=0  Vf=0  IC=0  UseSnubber=off  Rs=1e4  Cs=250e-9  Measurements=off
  IGBT1 : powerlib/Power Electronics/IGBT  DialogController=POWERSYS.PowerSysDialog  SystemSampleTime=-1  Ron=0.001  Lon=0  Vf=1  Tf=1e-6  Tt=2e-6  IC=0  Rs=1e5  Cs=inf  Measurements=off
  IGBT2 : powerlib/Power Electronics/IGBT  DialogController=POWERSYS.PowerSysDialog  SystemSampleTime=-1  Ron=0.001  Lon=0  Vf=1  Tf=1e-6  Tt=2e-6  IC=0  Rs=1e5  Cs=inf  Measurements=off
  + : PMIOPort  Port=1  Side=Left
  - : PMIOPort  Port=2  Side=Right
  wires:
  g/1 -> IGBT1/1, IGBT2/1
  connections:
  Diode1/LConn1 -- IGBT1/RConn1 -- IGBT2/RConn1 -- Diode/LConn1
  Diode1/RConn1 -- IGBT1/LConn1 -- -/RConn1
  Diode/RConn1 -- IGBT2/LConn1 -- +/RConn1
